simulink model "AOOVOOswitch"  (R2023b)
settings: Solver=FixedStepAuto  StartTime=0.0  StopTime=10  FixedStep=1e-3  RelTol=1e-3  EnableMultiTasking=on
undefined symbols (not defined in the file or in its folder): D10, D11, D12, D2, D4, D7, D8, D9, PTA0, PTB23, PTB9, PTC3, PTC4, PTD0, PTD2, PTD3
libraries: frdmk64flib x8
settings Model: PacingRate=0.250000  ExtModeTrigDuration=5  Creator=mathewgaluszka  LastModifiedBy=mathewgaluszka
settings OptimizationCC: EnhancedBackFolding=on  PassReuseOutputArgsAs=Individual arguments  ZeroExternalMemoryAtStartup=off  ZeroInternalMemoryAtStartup=off  MaxStackSize=64  OptimizeBlockOrder=speed  DifferentSizesBufferReuse=on  OptimizationCustomize=off  EfficientTunableParamExpr=on
settings DebuggingCC: ParameterTunabilityLossMsg=error
settings HardwareCC: ProdBitPerPointer=32  ProdBitPerSizeT=32  ProdBitPerPtrDiffT=32  ProdLargestAtomicInteger=Long  ProdLargestAtomicFloat=Double  ProdWordSize=32  ProdHWDeviceType=ARM Compatible->ARM Cortex
settings SFSimCC: MATLABDynamicMemAlloc=off
settings RTWCC: Description=Embedded Coder  SystemTargetFile=ert.tlc  HardwareBoard=NXP FRDM-K64F  TLCOptions="-aInlineSetEventsForThisBaseRateFcn=TLC_FALSE -aSuppressMultiTaskScheduler=TLC_FALSE  -aRateBasedStepFcn=0"  TemplateMakefile=ert_default_tmf  Toolchain=GNU Tools for ARM Embedded Processors
settings CodeAppCC: ForceParamTrailComments=on  IgnoreCustomStorageClasses=off  OperatorAnnotations=on  SimulinkDataObjDesc=on  SFDataObjDesc=on  InsertBlockDesc=on
settings ERTTargetCC: ExtModeTransport=4  ExtModeMexFile=sendToCommService

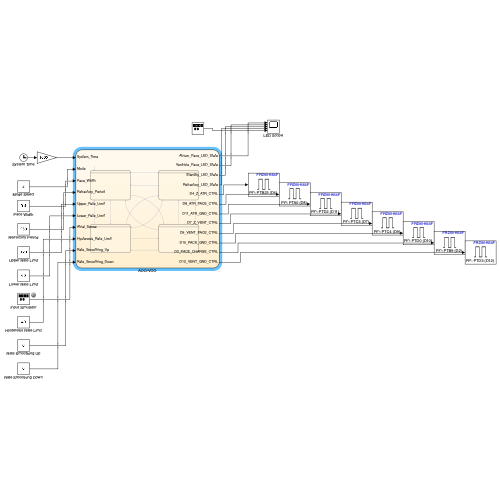
[thumbnail: Simulink's stored preview of the top-level diagram]
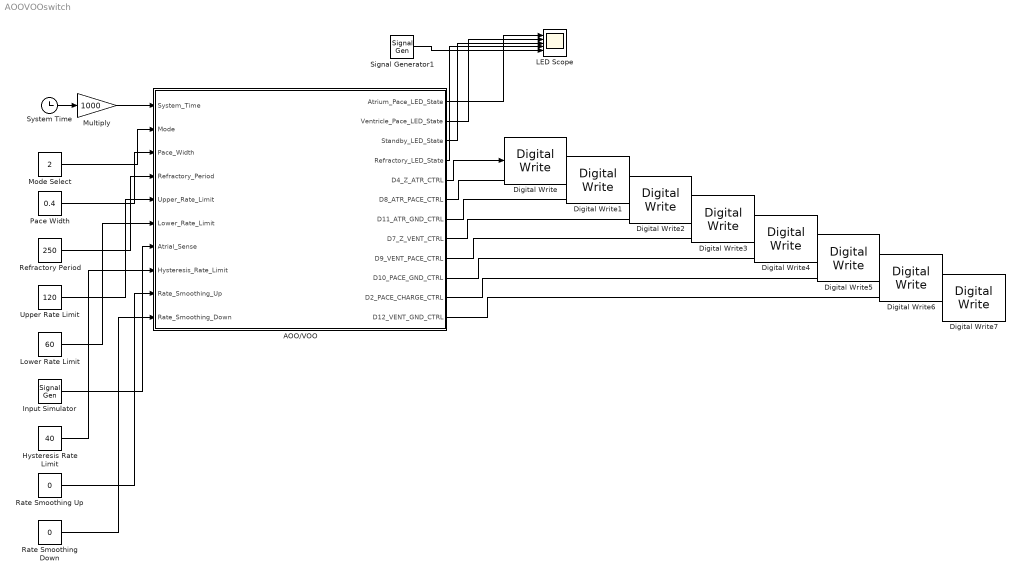
== system AOOVOOswitch ==
  AOO/VOO : Stateflow chart  TreatAsAtomicUnit=on
  Digital Write : frdmk64flib/Digital Write  Whichpin=PTB23 (D4)
  Digital Write1 : frdmk64flib/Digital Write  Whichpin=PTA0 (D8)
  Digital Write2 : frdmk64flib/Digital Write  Whichpin=PTD2 (D11)
  Digital Write3 : frdmk64flib/Digital Write  Whichpin=PTC3 (D7)
  Digital Write4 : frdmk64flib/Digital Write  Whichpin=PTC4 (D9)
  Digital Write5 : frdmk64flib/Digital Write  Whichpin=PTD0 (D10)
  Digital Write6 : frdmk64flib/Digital Write  Whichpin=PTB9 (D2)
  Digital Write7 : frdmk64flib/Digital Write  Whichpin=PTD3 (D12)
  Hysteresis Rate Limit : Constant  Value=40
  Input Simulator : SignalGenerator  WaveForm=sawtooth
  LED Scope : Scope  NumInputPorts=5
  Lower Rate Limit : Constant  Value=60
  Mode Select : Constant  Value=2
  Multiply : Gain  Gain=1000
  Pace Width : Constant  Value=0.4
  Rate Smoothing Down : Constant  Value=0
  Rate Smoothing Up : Constant  Value=0
  Refractory Period : Constant  Value=250
  Signal Generator1 : SignalGenerator  WaveForm=sawtooth
  System Time : Clock
  Upper Rate Limit : Constant  Value=120
  wires:
  Mode Select/1 -> AOO/VOO/2(Mode)
  Pace Width/1 -> AOO/VOO/3(Pace_Width)
  Refractory Period/1 -> AOO/VOO/4(Refractory_Period)
  AOO/VOO/1(Atrium_Pace_LED_State) -> LED Scope/1
  AOO/VOO/2(Ventricle_Pace_LED_State) -> LED Scope/2
  Upper Rate Limit/1 -> AOO/VOO/5(Upper_Rate_Limit)
  Lower Rate Limit/1 -> AOO/VOO/6(Lower_Rate_Limit)
  AOO/VOO/3(Standby_LED_State) -> LED Scope/3
  AOO/VOO/5(D4_Z_ATR_CTRL) -> Digital Write/1
  AOO/VOO/6(D8_ATR_PACE_CTRL) -> Digital Write1/1
  AOO/VOO/7(D11_ATR_GND_CTRL) -> Digital Write2/1
  AOO/VOO/8(D7_Z_VENT_CTRL) -> Digital Write3/1
  AOO/VOO/9(D9_VENT_PACE_CTRL) -> Digital Write4/1
  AOO/VOO/10(D10_PACE_GND_CTRL) -> Digital Write5/1
  AOO/VOO/11(D2_PACE_CHARGE_CTRL) -> Digital Write6/1
  AOO/VOO/12(D12_VENT_GND_CTRL) -> Digital Write7/1
  AOO/VOO/4(Refractory_LED_State) -> LED Scope/4
  Input Simulator/1 -> AOO/VOO/7(Atrial_Sense)
  Hysteresis Rate Limit/1 -> AOO/VOO/8(Hysteresis_Rate_Limit)
  Signal Generator1/1 -> LED Scope/5
  Rate Smoothing Up/1 -> AOO/VOO/9(Rate_Smoothing_Up)
  Rate Smoothing Down/1 -> AOO/VOO/10(Rate_Smoothing_Down)
  System Time/1 -> Multiply/1
  Multiply/1 -> AOO/VOO/1(System_Time)

== stateflow chart AOOVOOswitch/AOO//VOO ==
  state AOO
    state Pace
      entry:
      Atrium_Pace_LED_State=true;
      Standby_LED_State=false;
      D2_PACE_CHARGE_CTRL=0;
      D10_PACE_GND_CTRL=1;
      D8_ATR_PACE_CTRL=1;
      D11_ATR_GND_CTRL=0;
      D4_Z_ATR_CTRL=0;
      D7_Z_VENT_CTRL=0;
      D12_VENT_GND_CTRL=0;
      D9_VENT_PACE_CTRL=0;
    state Standby
      entry:
      Atrium_Pace_LED_State=false;
      Standby_LED_State=true;
      D10_PACE_GND_CTRL=1;
      D9_VENT_PACE_CTRL=0;
      D4_Z_ATR_CTRL=0;
      D7_Z_VENT_CTRL=0;
      D8_ATR_PACE_CTRL=0;
      D11_ATR_GND_CTRL=1;
      D12_VENT_GND_CTRL=0;
      D2_PACE_CHARGE_CTRL=1;
      Standby_Period=(1/(Lower_Rate_Limit))*60000
    (default) -> AOO.Standby
    AOO.Pace -> AOO.Standby : [after(Pace_Width,msec)]
    AOO.Standby -> AOO.Pace : [after(Standby_Period,msec)]
  state AAI
    state Pace
      entry:
      Hysteresis_State=false;
      Atrium_Pace_LED_State=true;
      Standby_LED_State=false;
      Refractory_LED_State=false;
      D2_PACE_CHARGE_CTRL=0;
      D10_PACE_GND_CTRL=1;
      D8_ATR_PACE_CTRL=1;
      D11_ATR_GND_CTRL=0;
      D4_Z_ATR_CTRL=0;
      D7_Z_VENT_CTRL=0;
      D12_VENT_GND_CTRL=0;
      D9_VENT_PACE_CTRL=0;
    state Refractory
      entry:
      Atrium_Pace_LED_State=false;
      Standby_LED_State=false;
      Refractory_LED_State=true;
      D10_PACE_GND_CTRL=1;
      D9_VENT_PACE_CTRL=0;
      D4_Z_ATR_CTRL=0;
      D7_Z_VENT_CTRL=0;
      D8_ATR_PACE_CTRL=0;
      D11_ATR_GND_CTRL=1;
      D12_VENT_GND_CTRL=0;
      D2_PACE_CHARGE_CTRL=1;
    state Entry
      entry:
      Hysteresis_State=false;
    state Natural_Pace
      entry:
      Prev_Standby_Period=System_Time-Start_Time;
      Atrium_Pace_LED_State=true;
      Hysteresis_State=true;
    state Standby_Select
      state Standby
        entry:
        Atrium_Pace_LED_State=false;
        Standby_LED_State=true;
        Refractory_LED_State=false;
        Standby_Period = (1/(Lower_Rate_Limit))*60000-Refractory_Period;
      state Greater
        entry:
        Standby_Period=(Prev_Standby_Period+Refractory_Period)*(1+1/100*(Rate_Smoothing_Up))-Refractory_Period;
      state Entry
        entry:
        Start_Time=System_Time;
      state Rate_Smoothing_Active
      state Exit
        exit:
        Prev_Standby_Period=System_Time-Start_Time
      state Standby_Hysteresis
        entry:
        Atrium_Pace_LED_State=false;
        Standby_LED_State=true;
        Refractory_LED_State=false;
        Standby_Period = (1/(Hysteresis_Rate_Limit))*60000-Refractory_Period;
      state Less
        entry:
        Standby_Period=(Prev_Standby_Period+Refractory_Period)*(1-1/100*(Rate_Smoothing_Down))-Refractory_Period;
      AAI.Standby_Select.Standby -> Exit [order 2]
      AAI.Standby_Select.Entry -> AAI.Standby_Select.Standby [order 1] : [Hysteresis_State==false]
      Rate_Smoothing_Active -> Greater [order 1] : [(Standby_Period+Refractory_Period)>(Prev_Standby_Period+Refractory_Period)*(1+1/100*(Rate_Smoothing_Up))]
      Greater -> Exit
      AAI.Standby_Select.Standby -> Rate_Smoothing_Active [order 1] : [(Rate_Smoothing_Up~=0)||(Rate_Smoothing_Down~=0)]
      (default) -> AAI.Standby_Select.Entry
      Standby_Hysteresis -> Rate_Smoothing_Active [order 1] : [(Rate_Smoothing_Up~=0)||(Rate_Smoothing_Down~=0)]
      Rate_Smoothing_Active -> Less [order 2] : [(Standby_Period+Refractory_Period)<(Prev_Standby_Period+Refractory_Period)*(1-1/100*(Rate_Smoothing_Down))]
      AAI.Standby_Select.Entry -> Standby_Hysteresis [order 2] : [Hysteresis_State==true]
      Standby_Hysteresis -> Exit [order 2]
      Less -> Exit
    (default) -> AAI.Entry
    AAI.Pace -> Refractory : [after(Pace_Width,msec)]
    AAI.Entry -> Refractory
    Natural_Pace -> Refractory
    Standby_Select -> Natural_Pace [order 2] : [Atrial_Sense==1]
    Refractory -> Standby_Select : [after(Refractory_Period,msec)]
    Standby_Select -> AAI.Pace [order 1] : [after(Standby_Period,msec)]
  state VOO
    state Pace
      entry:
      Ventricle_Pace_LED_State=true;
      Standby_LED_State=false;
      D2_PACE_CHARGE_CTRL=0;
      D10_PACE_GND_CTRL=1;
      D8_ATR_PACE_CTRL=0;
      D11_ATR_GND_CTRL=0;
      D4_Z_ATR_CTRL=0;
      D7_Z_VENT_CTRL=0;
      D12_VENT_GND_CTRL=0;
      D9_VENT_PACE_CTRL=1;
    state Standby
      entry:
      Ventricle_Pace_LED_State=false;
      Standby_LED_State=true;
      D10_PACE_GND_CTRL=1;
      D9_VENT_PACE_CTRL=0;
      D4_Z_ATR_CTRL=0;
      D7_Z_VENT_CTRL=0;
      D8_ATR_PACE_CTRL=0;
      D11_ATR_GND_CTRL=0;
      D12_VENT_GND_CTRL=1;
      D2_PACE_CHARGE_CTRL=1;
      Standby_Period=(1/(Lower_Rate_Limit))*60000
    (default) -> VOO.Standby
    VOO.Pace -> VOO.Standby : [after(Pace_Width,msec)]
    VOO.Standby -> VOO.Pace : [after(Standby_Period,msec)]
  state VVI
  (default) -> AOO
  AOO -> AAI [order 1] : [Mode==2]
  AAI -> AOO [order 2] : [Mode==0]
  AOO -> VVI [order 3] : [Mode==3]
  VOO -> AAI [order 3] : [Mode==2]
  VOO -> AOO [order 1] : [Mode==0]
  AOO -> VOO [order 2] : [Mode==1]
  VVI -> AOO [order 3] : [Mode==0]
  AAI -> VOO [order 3] : [Mode==1]
  VVI -> AAI [order 2] : [Mode==2]
  AAI -> VVI [order 1] : [Mode==3]
  VOO -> VVI [order 2] : [Mode==3]
  VVI -> VOO [order 1] : [Mode==1]
  data: System_Time input; Mode input; Pace_Width input; Refractory_Period input; Atrium_Pace_LED_State output; Ventricle_Pace_LED_State output; Standby_LED_State output; Refractory_LED_State output; D4_Z_ATR_CTRL output; D8_ATR_PACE_CTRL output; D11_ATR_GND_CTRL output; D7_Z_VENT_CTRL output; D9_VENT_PACE_CTRL output; D10_PACE_GND_CTRL output; D2_PACE_CHARGE_CTRL output; D12_VENT_GND_CTRL output; Upper_Rate_Limit input; Lower_Rate_Limit input; Standby_Period local; Atrial_Sense input; Hysteresis_State local; Hysteresis_Rate_Limit input; Prev_Standby_Period local; Rate_Smoothing_Up input; Rate_Smoothing_Down input; Start_Time local
